simulink model "Z5"  (R2017b)
settings: Solver=FixedStepAuto  StartTime=0.0  StopTime=100.0  FixedStep=0.001  RelTol=1e-3
values from neighbouring files (symbols this model uses):
  k = k+26    [Caesarcipher.m]
  m = mean(r)    [plotrand.m]
settings Model: Creator=Mahe  LastModifiedBy=Mahe

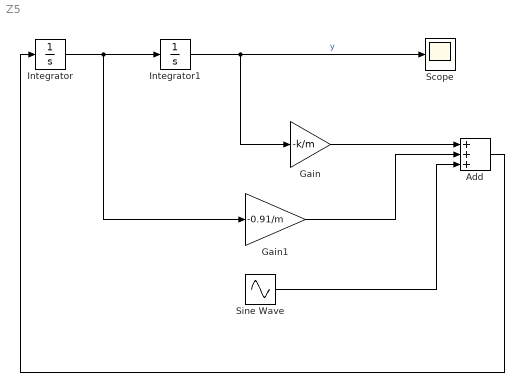
== system Z5 ==
  Add : Sum  Inputs=+++
  Gain : Gain  Gain=-k/m
  Gain1 : Gain  Gain=-0.91/m
  Integrator : Integrator
  Integrator1 : Integrator  InitialCondition=20
  Scope : Scope
  Sine Wave : Sin  Amplitude=10  Frequency=0.7073  Phase=pi/2  SampleTime=0
  wires:
  Integrator/1 -> Gain1/1, Integrator1/1
  Integrator1/1 -> Scope/1, Gain/1  "y"
  Gain/1 -> Add/1
  Gain1/1 -> Add/2
  Add/1 -> Integrator/1
  Sine Wave/1 -> Add/3
